simulink model "PendulumRobotDynamics"  (R2024a)
settings: Solver=ode3  StartTime=0.0  StopTime=20  FixedStep=0.002  RelTol=1e-3  EnableMultiTasking=on
libraries: quarc_library x2
settings Model: ExtModeTrigDuration=10000  Creator=schuster.t  LastModifiedBy=schuster.t
settings SolverCC: AlgebraicLoopSolver=TrustRegion  PositivePriorityOrder=on
settings DataIOCC: ReturnWorkspaceOutputs=off
settings DebuggingCC: UnconnectedInputMsg=warning  UnconnectedOutputMsg=warning  UnconnectedLineMsg=warning  ArithmeticOperatorsInVariantConditions=warning
settings ModelReferenceCC: EnableRefExpFcnMdlSchedulingChecks=on
settings SFSimCC: SimUseLocalCustomCode=off  CustomCodeUndefinedFunction=UseInterfaceOnly
settings RTWCC: Description=QUARC Win64 Target Using Toolchain  SystemTargetFile=quarc_win64.tlc  TemplateMakefile=quarc_default_tmf  RTWUseLocalCustomCode=off  Toolchain=QUARC win64 | nmake (64-bit Windows)  BuildConfiguration=Faster Runs  GPUComputeCapability=3.5
settings CodeAppCC: StateflowObjectComments=on
settings STFCustomTargetCC: ConcurrentExecutionCompliant=on  SystemTargetFile=quarc_win64.tlc
settings GRTTargetCC: ParMdlRefBuildCompliant=off  CompOptLevelCompliant=off  CombineOutputUpdateFcns=off  MatFileLogging=off  CPPClassGenCompliant=off  GRTInterface=on  ExtMode=on  ExtModeMexFile=quarc_comm
settings ConfigComp: CovMetricSettings=dswe

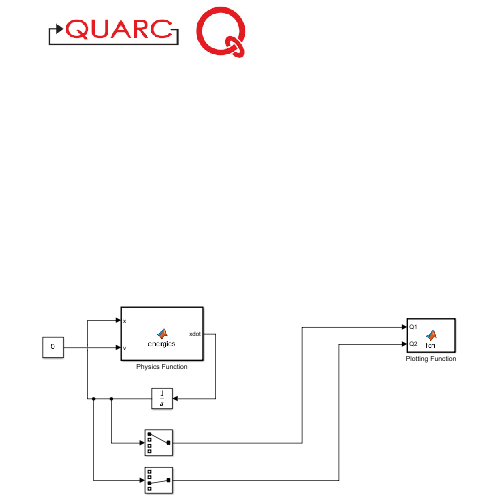
[thumbnail: Simulink's stored preview of the top-level diagram]
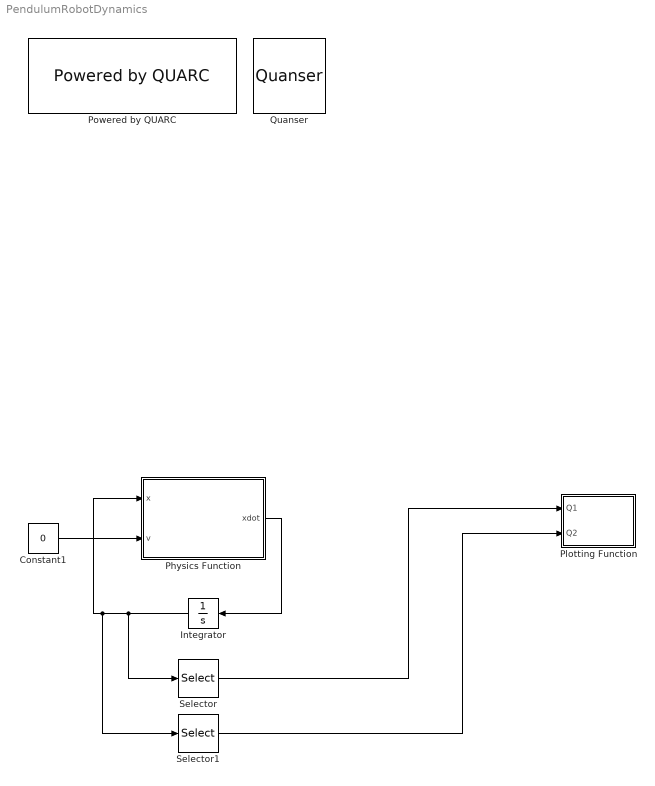
== system PendulumRobotDynamics ==
  Constant1 : Constant  Value=0
  Integrator : Integrator  InitialCondition=[0; 0; 0; 0]
  Physics Function : MATLAB Function  TreatAsAtomicUnit=on
  Plotting Function : MATLAB Function  TreatAsAtomicUnit=on
  Powered by QUARC : quarc_library/Logos/Powered by QUARC
  Quanser : quarc_library/Logos/Quanser
  Selector : Selector  InputPortWidth=4  IndexOptions=Index vector (dialog)  Indices=[1]  OutputSizes=1
  Selector1 : Selector  InputPortWidth=4  IndexOptions=Index vector (dialog)  Indices=[3]  OutputSizes=1
  wires:
  Physics Function/1(xdot) -> Integrator/1
  Integrator/1 -> Selector/1, Selector1/1, Physics Function/1(x)
  Constant1/1 -> Physics Function/2(v)
  Selector/1 -> Plotting Function/1(Q1)
  Selector1/1 -> Plotting Function/2(Q2)

== matlab function PendulumRobotDynamics/Physics Function ==
  data: x input; xdot output; v input
function xdot = energies(x, v)

    % Theta values
    theta1 = 0.0304;
    theta2 = 0.0184;
    theta3 = 0.0184;
    theta4 = 0.0921;
    theta5 = 0.6101;
    theta6 = 0.0097;

    % Energy matrices
    q1 = x(1);
    q1dot = x(2);
    q2 = x(3);
    q2dot = x(4);

    m11 = theta1+sin(q2)^2*theta2;
    m12 = theta3*cos(q2);
    m21 = theta3*cos(q2);
    m22 = theta2;
    m = [m11 m12; m21 m22];
    
    c11 = 2*theta2*sin(q2)*cos(q2)*q2dot;
    c12 = -theta3*sin(q2)*q2dot;
    c21 = -theta2*sin(q2)*cos(q2)*q1dot;
    c22 = 0;
    c = [c11 c12; c21 c22];

    f1 = theta5*q1dot;
    f2 = theta6*q2dot;
    f = [f1; f2];
    
    g1 = 0;
    g2 = -theta4*9.81*sin(q2);
    gMatrix = [g1; g2];

    qdotdot = m^-1 * ([v; 0] - (c*[q1dot; q2dot]+f+gMatrix));

    xdot = [q1dot; qdotdot(1); q2dot; qdotdot(2)];

== matlab function PendulumRobotDynamics/Plotting Function ==
  data: Q1 input; Q2 input
function fcn(Q1, Q2)
    hold on
    grid on
    axis([-20 20 -20 20 -5 15]);
    view(3)
    BaseDesX = [0, 0];
    BaseDesY = [0, 0];
    BaseDesZ = [-5, 0];
    plot3(BaseDesX,BaseDesY,BaseDesZ,'rs-', 'LineWidth', 2, 'MarkerSize', 8);

    theta1 = Q1;
    transformLink1(theta1);
    theta2 = Q2;
    transformLink2(theta1, theta2);  

end
